simulink model "Hinf_BS_Comparison"  (R2026a)
settings: Solver=ode23tb  StopTime=175  FixedStep=0.0001  MaxStep=0.02  RelTol=1e-9  AbsTol=1e-12
PostLoadFcn:
  | init_comparison(bdroot);
InitFcn:
  | init_comparison(bdroot);
model workspace (MAT data in the model file):
  A = [-4.33427458178e-18 -1739.27628419 -1.9879507565e-12 -947.702562069 9.25490783271 -3.87188490855e-14 40.5994463199 -1.82279284791e-15 1.34368571874e-07 -8.90717137351e-10 -711.607566004 -711.607566004 ... (196 elements, 14x14)]
  B = [-1.75563782385e-19; 2.23785567073e-19; -10165.2431057; -49.2726170531; 5.13589910552; -5.90943945895; 6.81435391425; 45.4160051294; 1073741824; 17236611.4468; 7.60467680903e-16; -1.03174259462e-14; 5.13319473105e-15; 5.73530096059e-15]
  C = [-313107.329042 -2686499.93691 37750.0108104 101565.096764 -37.2177294622 -2820.69827595 3048.09156473 3382.76066655 -2.10142044744 -107.98720369 -2843187.08558 -2796371.67099 -2071651.86494 -912132.974279]
  D = 0
  a1 = 3
  a2 = 3
  a3 = 3
  a4 = 3
  b = -100
  k1 = 9.81
  k1_0 = 9.81
  k1_3 = 7.3575
  k2 = 0.555555555556
  k2_0 = 1.11111111111
  k2_3 = 6.66666666667
  k3 = 2.9
  k3_0 = 2
  k3_3 = 7.93333333333
  k4 = 1.8
  k4_0 = 0.9
  k4_3 = 0.45
  k5 = 0.620689655172
  k5_0 = 0.45
  k5_3 = 0.0567226890756
  r_test = [0 0.02 0.04 0.06 0.08 0.1 0.12 0.14 0.16 0.18 0.2 0.22 ... (17570 elements, 8785x2)]
  w = 500
(part 1 of 2)
settings Model: Creator=bkurkcu  LastModifiedBy=bkurkcu

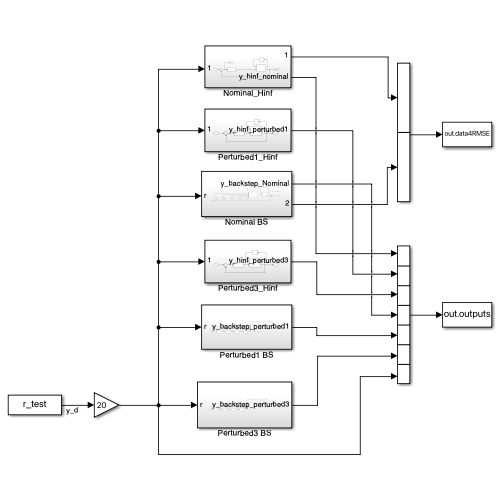
[thumbnail: Simulink's stored preview of the top-level diagram]
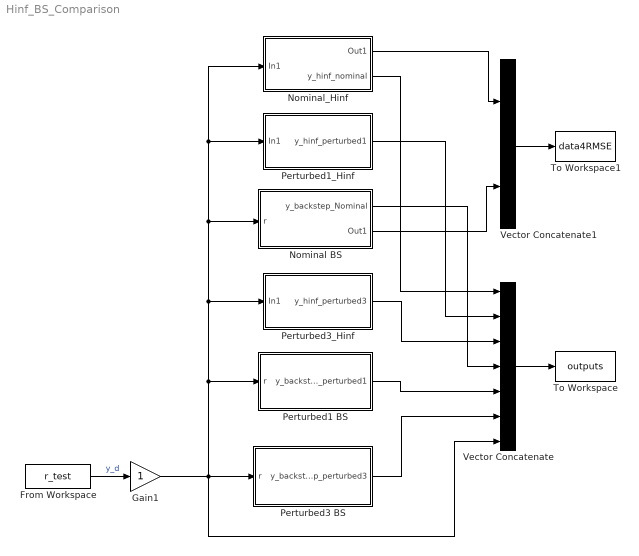
== system Hinf_BS_Comparison ==
  From Workspace : FromWorkspace  VariableName=r_test
  Gain1 : Gain
  Nominal BS : Subsystem
  Nominal_Hinf : Subsystem
  Perturbed1 BS : Subsystem
  Perturbed1_Hinf : Subsystem
  Perturbed3 BS : Subsystem
  Perturbed3_Hinf : Subsystem
  To Workspace : ToWorkspace  VariableName=outputs  SaveFormat=Structure With Time  SampleTime=0.001
  To Workspace1 : ToWorkspace  VariableName=data4RMSE  SaveFormat=Structure With Time  SampleTime=0.001
  Vector Concatenate : Concatenate  NumInputs=7
  Vector Concatenate1 : Concatenate
  wires:
  Vector Concatenate/1 -> To Workspace/1
  Vector Concatenate1/1 -> To Workspace1/1
  Perturbed3 BS/1(y_backstep_perturbed3) -> Vector Concatenate/6
  Perturbed3_Hinf/1(y_hinf_perturbed3) -> Vector Concatenate/3
  Perturbed1 BS/1(y_backstep_perturbed1) -> Vector Concatenate/5
  Nominal BS/2(Out1) -> Vector Concatenate1/2
  Perturbed1_Hinf/1(y_hinf_perturbed1) -> Vector Concatenate/2
  Nominal BS/1(y_backstep_Nominal) -> Vector Concatenate/4
  From Workspace/1 -> Gain1/1  "y_d"
  Nominal_Hinf/2(y_hinf_nominal) -> Vector Concatenate/1
  Nominal_Hinf/1(Out1) -> Vector Concatenate1/1
  Gain1/1 -> Perturbed3 BS/1(r), Vector Concatenate/7, Nominal BS/1(r), Nominal_Hinf/1(In1), Perturbed1_Hinf/1(In1), Perturbed3_Hinf/1(In1), Perturbed1 BS/1(r)
